simulink model "inclass_0923"  (R2025b)
settings: Solver=VariableStepAuto  StartTime=0.0  StopTime=10.0  RelTol=1e-3
settings Model: Creator=sprinkle  LastModifiedBy=sprinkle

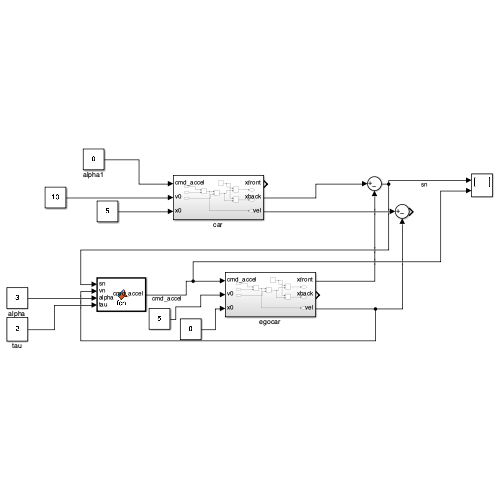
[thumbnail: Simulink's stored preview of the top-level diagram]
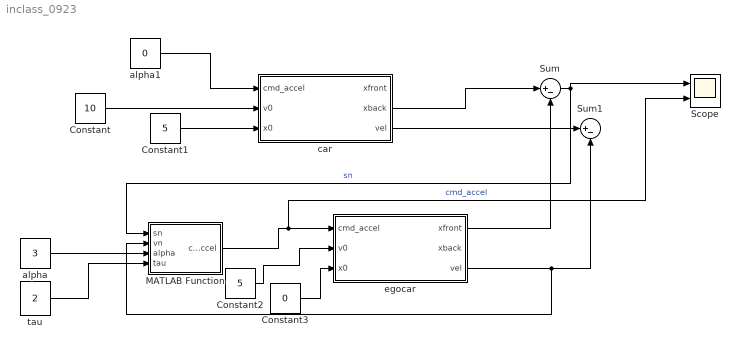
== system inclass_0923 ==
  Constant : Constant  Value=10
  Constant1 : Constant  Value=5
  Constant2 : Constant  Value=5
  Constant3 : Constant  Value=0
  MATLAB Function : MATLAB Function  TreatAsAtomicUnit=on
  Scope : Scope  NumInputPorts=2
      settings: ActiveDisplayYMinimum=-33.674641213079582  ActiveDisplayYMaximum=25.87177091771623
  Sum : Sum  Inputs=|+-
  Sum1 : Sum  Inputs=|+-
  alpha : Constant  Value=3
  alpha1 : Constant  Value=0
  car : Subsystem
  egocar : Subsystem
  tau : Constant  Value=2
  wires:
  car/2(xback) -> Sum/1
  egocar/1(xfront) -> Sum/2
  car/3(vel) -> Sum1/1
  egocar/3(vel) -> MATLAB Function/2(vn), Sum1/2
  MATLAB Function/1(cmd_accel) -> Scope/2, egocar/1(cmd_accel)  "cmd_accel"
  Sum/1 -> Scope/1, MATLAB Function/1(sn)  "sn"
  alpha/1 -> MATLAB Function/3(alpha)
  tau/1 -> MATLAB Function/4(tau)
  alpha1/1 -> car/1(cmd_accel)
  Constant1/1 -> car/3(x0)
  Constant/1 -> car/2(v0)
  Constant2/1 -> egocar/2(v0)
  Constant3/1 -> egocar/3(x0)

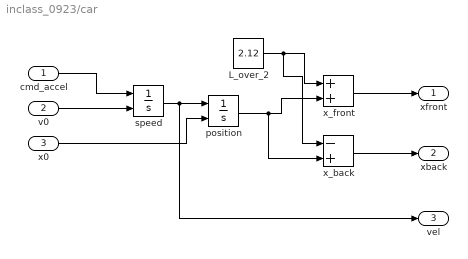
== system inclass_0923/car ==
  cmd_accel : Inport
  v0 : Inport  Port=2
  x0 : Inport  Port=3
  L_over_2 : Constant  Value=2.12
  position : Integrator  InitialConditionSource=external
  speed : Integrator  InitialConditionSource=external
  x_back : Sum  Inputs=-+
  x_front : Sum
  xfront : Outport
  xback : Outport  Port=2
  vel : Outport  Port=3
  wires:
  x_back/1 -> xback/1
  x0/1 -> position/2
  cmd_accel/1 -> speed/1
  speed/1 -> vel/1, position/1
  position/1 -> x_back/2, x_front/2
  x_front/1 -> xfront/1
  v0/1 -> speed/2
  L_over_2/1 -> x_back/1, x_front/1

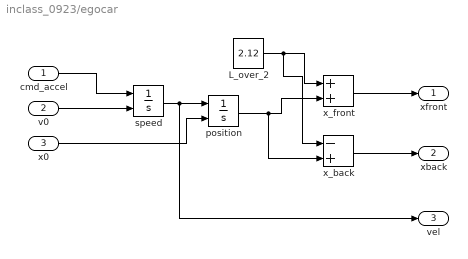
== system inclass_0923/egocar ==
  cmd_accel : Inport
  v0 : Inport  Port=2
  x0 : Inport  Port=3
  L_over_2 : Constant  Value=2.12
  position : Integrator  InitialConditionSource=external
  speed : Integrator  InitialConditionSource=external
  x_back : Sum  Inputs=-+
  x_front : Sum
  xfront : Outport
  xback : Outport  Port=2
  vel : Outport  Port=3
  wires:
  x_back/1 -> xback/1
  x0/1 -> position/2
  cmd_accel/1 -> speed/1
  speed/1 -> vel/1, position/1
  position/1 -> x_back/2, x_front/2
  x_front/1 -> xfront/1
  v0/1 -> speed/2
  L_over_2/1 -> x_back/1, x_front/1

== matlab function inclass_0923/MATLAB Function ==
  data: sn input; cmd_accel output; vn input; alpha input; tau input
function cmd_accel = fcn(sn,vn, alpha, tau)

cmd_accel = alpha * ( sn - tau * vn);
